simulink model "Problem17_model_v2"  (R2020b)
settings: Solver=ode4  StartTime=0.0  StopTime=SIM_TIME  FixedStep=STEP_SIZE  RelTol=1e-3
values from neighbouring files (symbols this model uses):
  a4 = 0.98    [Problem7_9.m]    (also in calc_h.m; problem13.m; problem16.m; problem17.m)
  d1 = 1.5    [calc_h.m]    (also in problem17.m; problem18.m; problem20.m; problem21.m)
  feff = 2.4*10^(-5)    (= 2.4e-05)    [problem12.m]    (also in problem13.m; problem15.m; problem16.m; problem17.m)
  Jeff = 1/n^2 .* supD + J_M    [Problem7_9.m]    (also in problem12.m = [0.0188, 0.0188, 0.0027, 0.0004].'; problem13.m = [0.0188, 0.0188, 0.0027, 0.0004].'; problem15.m = [0.0188, 0.0188, 0.0027, 0.0004].'; problem16.m = [0.0188, 0.0188, 0.0027, 0.0004].')
  K_D = 2*zeta/omega_n * K_p - feff / kT    [problem12.m]    (also in problem13.m; problem15.m = (2*omega_n*zeta*tau_i + 1 - feff) ./ kT; problem16.m = (2*omega_n*zeta*tau_i + 1 - feff) ./ kT; problem17.m = (2*omega_n*zeta*tau_i + 1 - feff) ./ kT)
  K_I = omega_n^2 / kT * ones(4,1)    [problem15.m]    (also in problem16.m; problem17.m; problem18.m; problem20.m = omega_n^2 / kT .* ones(4,1))
  K_p = omega_n^2 * Jeff / kT    [problem12.m]    (also in problem13.m; problem15.m = (omega_n.^2*tau_i + 2*omega_n*zeta) ./ kT; problem16.m = (omega_n.^2*tau_i + 2*omega_n*zeta) ./ kT; problem17.m = (omega_n.^2*tau_i + 2*omega_n*zeta) ./ kT)
  kT = 0.17    [problem12.m]    (also in problem13.m; problem15.m; problem16.m; problem17.m)
  n = 53    [Problem7_9.m]    (also in Problem8_script.m = length(t); problem12.m; problem13.m; problem15.m)
  T_L = abs(h)    [problem13.m]    (also in problem15.m; problem16.m = zeros(4,1); problem17.m; problem18.m)
settings Model: Creator=Theis  LastModifiedBy=Theis

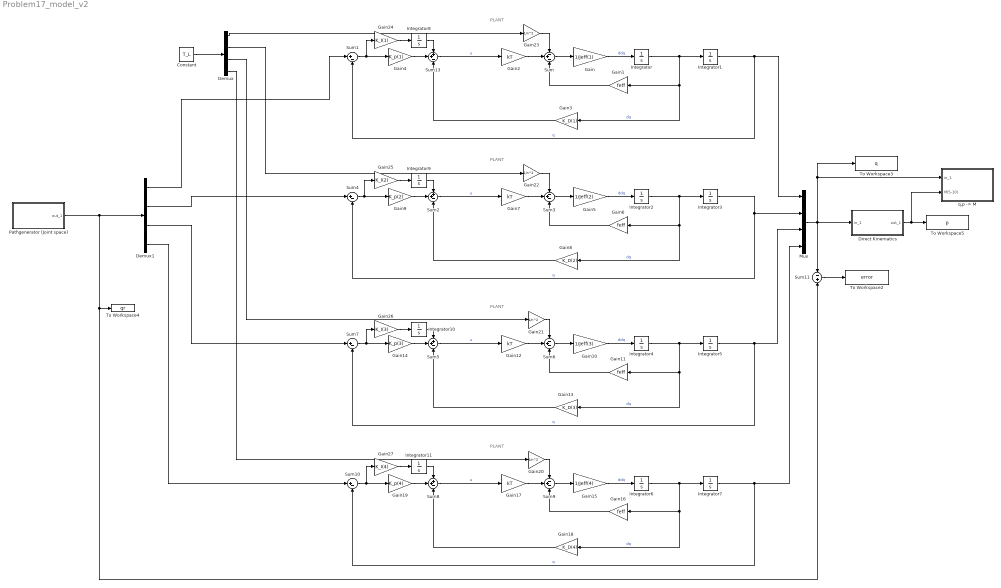
== system Problem17_model_v2 ==
  note: PLANT
  note: PLANT
  note: PLANT
  note: PLANT
  Constant : Constant  Value=T_L
  Demux : Demux
  Demux1 : Demux
  Direct Kinematics : Subsystem
      mask Display: disp('Alto-Robot')
  Gain : Gain  Gain=1/Jeff(1)
  Gain{1,6,11,16} (4 alike) : Gain  Gain=feff
  Gain10 : Gain  Gain=1/Jeff(3)
  Gain{2,7,12,17} (4 alike) : Gain  Gain=kT
  Gain13 : Gain  Gain=K_D(3)
  Gain14 : Gain  Gain=K_p(3)
  Gain15 : Gain  Gain=1/Jeff(4)
  Gain18 : Gain  Gain=K_D(4)
  Gain19 : Gain  Gain=K_p(4)
  Gain{20..23} (4 alike) : Gain  Gain=1/n^2
  Gain24 : Gain  Gain=K_I(1)
  Gain25 : Gain  Gain=K_I(2)
  Gain26 : Gain  Gain=K_I(3)
  Gain27 : Gain  Gain=K_I(4)
  Gain3 : Gain  Gain=K_D(1)
  Gain4 : Gain  Gain=K_p(1)
  Gain5 : Gain  Gain=1/Jeff(2)
  Gain8 : Gain  Gain=K_D(2)
  Gain9 : Gain  Gain=K_p(2)
  Integrator{,1..11} (12 alike) : Integrator
  Mux : Mux
  Pathgenerator (Joint space) : Subsystem
      mask Display: disp('Alto-Robot\n path -> q')
  Sum{,3,6,9} (4 alike) : Sum  Inputs=-+-
  Sum{1,4,7,10} (4 alike) : Sum  Inputs=|+-
  Sum11 : Sum  Inputs=-|+
  Sum{2,5,8,13} (4 alike) : Sum  Inputs=++-
  To Workspace2 : ToWorkspace  VariableName=error  SaveFormat=Timeseries  SampleTime=-1
  To Workspace3 : ToWorkspace  VariableName=q  SaveFormat=Timeseries  SampleTime=-1
  To Workspace4 : ToWorkspace  VariableName=qr
      settings: MaxDataPoints=10000
  To Workspace5 : ToWorkspace  VariableName=p  SaveFormat=Timeseries  SampleTime=-1
  "q,p -> M" : Subsystem
      mask Display: disp('Save to vis4link')
  wires:
  Integrator/1 -> Integrator1/1, Gain3/1, Gain1/1  "dq"
  Gain/1 -> Integrator/1  "ddq"
  Sum/1 -> Gain/1
  Sum13/1 -> Gain2/1  "u"
  Integrator1/1 -> Mux/1, Sum1/2  "q"
  Gain3/1 -> Sum13/3
  Sum1/1 -> Gain24/1, Gain4/1
  Gain4/1 -> Sum13/2
  Gain6/1 -> Sum3/3
  Gain7/1 -> Sum3/2
  Gain8/1 -> Sum2/3
  Gain9/1 -> Sum2/2
  Sum2/1 -> Gain7/1  "u"
  Sum3/1 -> Gain5/1
  Gain5/1 -> Integrator2/1  "ddq"
  Integrator2/1 -> Integrator3/1, Gain8/1, Gain6/1  "dq"
  Integrator3/1 -> Mux/2, Sum4/2  "q"
  Gain13/1 -> Sum5/3
  Sum5/1 -> Gain12/1  "u"
  Sum6/1 -> Gain10/1
  Integrator4/1 -> Integrator5/1, Gain13/1, Gain11/1  "dq"
  Gain10/1 -> Integrator4/1  "ddq"
  Integrator7/1 -> Mux/4, Sum10/2  "q"
  Gain14/1 -> Sum5/2
  Gain12/1 -> Sum6/2
  Integrator6/1 -> Integrator7/1, Gain18/1, Gain16/1  "dq"
  Sum9/1 -> Gain15/1
  Gain15/1 -> Integrator6/1  "ddq"
  Gain18/1 -> Sum8/3
  Sum8/1 -> Gain17/1  "u"
  Integrator5/1 -> Mux/3, Sum7/2  "q"
  Gain17/1 -> Sum9/2
  Gain16/1 -> Sum9/3
  Gain19/1 -> Sum8/2
  Gain11/1 -> Sum6/3
  Gain1/1 -> Sum/3
  Gain2/1 -> Sum/2
  Gain20/1 -> Sum9/1
  Gain21/1 -> Sum6/1
  Gain22/1 -> Sum3/1
  Gain23/1 -> Sum/1
  Constant/1 -> Demux/1
  Demux/1 -> Gain23/1
  Demux/2 -> Gain22/1
  Demux/3 -> Gain21/1
  Demux/4 -> Gain20/1
  Gain24/1 -> Integrator8/1
  Integrator8/1 -> Sum13/1
  Integrator9/1 -> Sum2/1
  Gain25/1 -> Integrator9/1
  Sum4/1 -> Gain25/1, Gain9/1
  Integrator10/1 -> Sum5/1
  Gain26/1 -> Integrator10/1
  Sum7/1 -> Gain26/1, Gain14/1
  Integrator11/1 -> Sum8/1
  Gain27/1 -> Integrator11/1
  Sum10/1 -> Gain27/1, Gain19/1
  Demux1/1 -> Sum1/1
  Demux1/2 -> Sum4/1
  Demux1/3 -> Sum7/1
  Demux1/4 -> Sum10/1
  Sum11/1 -> To Workspace2/1
  Mux/1 -> Direct Kinematics/1(in_1), Sum11/1, "q,p -> M"/1(in_1), To Workspace3/1
  Pathgenerator (Joint space)/1(out_1) -> Sum11/2, To Workspace4/1, Demux1/1
  Direct Kinematics/1(out_1) -> "q,p -> M"/2(M(5-10)), To Workspace5/1

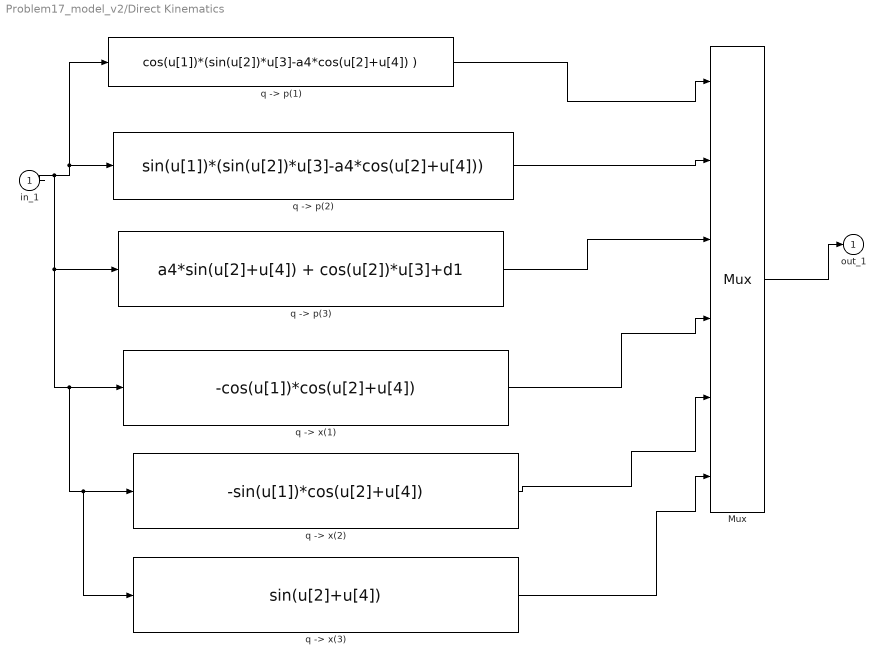
== system Problem17_model_v2/Direct Kinematics ==
  in_1 : Inport
  Mux : Mux  Inputs=6
  "q -> p(1)" : Fcn  Expr=cos(u[1])*(sin(u[2])*u[3]-a4*cos(u[2]+u[4]) )
  "q -> p(2)" : Fcn  Expr=sin(u[1])*(sin(u[2])*u[3]-a4*cos(u[2]+u[4]))
  "q -> p(3)" : Fcn  Expr=a4*sin(u[2]+u[4]) + cos(u[2])*u[3]+d1
  "q -> x(1)" : Fcn  Expr=-cos(u[1])*cos(u[2]+u[4])
  "q -> x(2)" : Fcn  Expr=-sin(u[1])*cos(u[2]+u[4])
  "q -> x(3)" : Fcn  Expr=sin(u[2]+u[4])
  out_1 : Outport  InitialOutput=0  VectorParamsAs1DForOutWhenUnconnected=off
  wires:
  Mux/1 -> out_1/1
  in_1/1 -> "q -> x(3)"/1, "q -> x(2)"/1, "q -> x(1)"/1, "q -> p(3)"/1, "q -> p(2)"/1, "q -> p(1)"/1
  "q -> x(3)"/1 -> Mux/6
  "q -> x(2)"/1 -> Mux/5
  "q -> x(1)"/1 -> Mux/4
  "q -> p(1)"/1 -> Mux/1
  "q -> p(2)"/1 -> Mux/2
  "q -> p(3)"/1 -> Mux/3

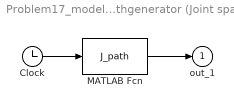
== system Problem17_model_v2/Pathgenerator (Joint space) ==
  Clock : Clock
  MATLAB Fcn : MATLABFcn  MATLABFcn=J_path  OutputDimensions=4
  out_1 : Outport  VectorParamsAs1DForOutWhenUnconnected=off
  wires:
  MATLAB Fcn/1 -> out_1/1
  Clock/1 -> MATLAB Fcn/1

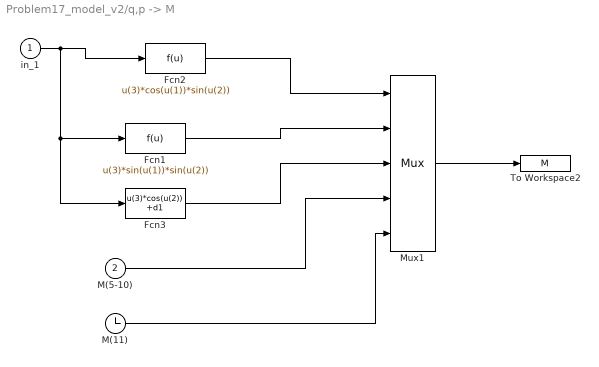
== system Problem17_model_v2/q,p -> M ==
  in_1 : Inport
  M(5-10) : Inport  Port=2
  Fcn1 : Fcn  Expr=u(3)*sin(u(1))*sin(u(2))
  Fcn2 : Fcn  Expr=u(3)*cos(u(1))*sin(u(2))
  Fcn3 : Fcn  Expr=u(3)*cos(u(2)) +d1
  M(11) : Clock
  Mux1 : Mux  Inputs=[1 1 1 6 1]
  To Workspace2 : ToWorkspace  VariableName=M
      settings: MaxDataPoints=100000
  wires:
  M(11)/1 -> Mux1/5
  M(5-10)/1 -> Mux1/4
  Fcn3/1 -> Mux1/3
  Fcn1/1 -> Mux1/2
  Fcn2/1 -> Mux1/1
  in_1/1 -> Fcn3/1, Fcn1/1, Fcn2/1
  Mux1/1 -> To Workspace2/1
